simulink model "PTC_MBDS_TurnOnDelaySample_Sample"  (R2013a)
settings: Solver=FixedStepDiscrete  StartTime=0.0  StopTime=100  FixedStep=Auto  RelTol=1e-3
undefined symbols (not defined in the file): sigbuilder_block
libraries: simulink_extras x1, PTC_MBDS_LIB x1
settings Model: Creator=uidl7367  LastModifiedBy=sundeep.tuteja
settings DataIOCC: SignalLoggingSaveFormat=ModelDataLogs
settings OptimizationCC: ExpressionDepthLimit=2147483647  InitFltsAndDblsToZero=on
settings DebuggingCC: SaveWithParameterizedLinksMsg=none  SignalResolutionControl=TryResolveAllWithWarning  SolverPrmCheckMsg=none  InheritedTsInSrcMsg=none  MultiTaskDSMMsg=warning  MultiTaskCondExecSysMsg=none  FcnCallInpInsideContextMsg=UseLocalSettings  StrictBusMsg=Warning
settings RTWCC: IncludeERTFirstTime=on
settings GRTTargetCC: TargetFcnLib=ansi_tfl_tmw.mat  CombineOutputUpdateFcns=off  GRTInterface=on

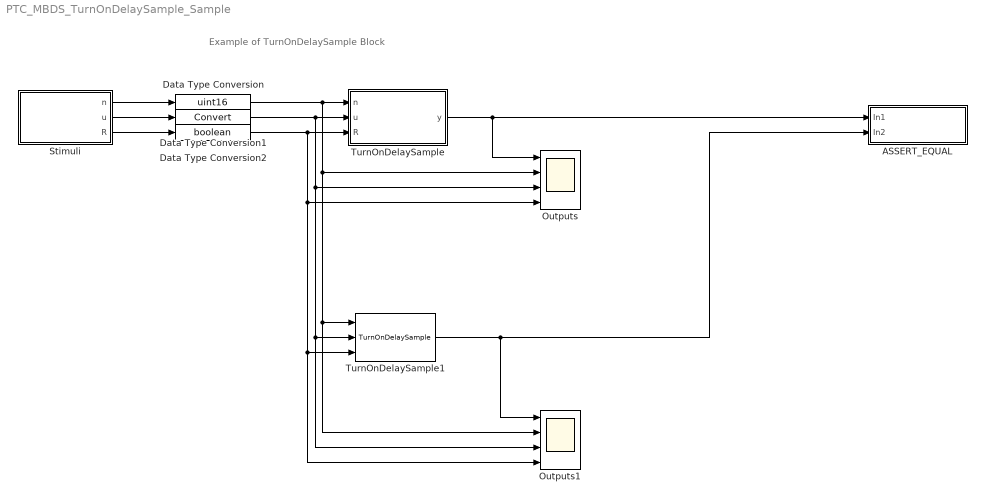
== system PTC_MBDS_TurnOnDelaySample_Sample ==
  note: Example of TurnOnDelaySample Block
  ASSERT_EQUAL : Subsystem
  Data Type Conversion : DataTypeConversion  InitFcn=|  OutDataTypeStr=uint16  SaturateOnIntegerOverflow=on
      | try
      |    MBDS_BlockCallback('Update', gcb);
      | end
  Data Type Conversion1 : DataTypeConversion  InitFcn=|  SaturateOnIntegerOverflow=on
      | try
      |    MBDS_BlockCallback('Update', gcb);
      | end
  Data Type Conversion2 : DataTypeConversion  InitFcn=|  OutDataTypeStr=boolean  SaturateOnIntegerOverflow=on
      | try
      |    MBDS_BlockCallback('Update', gcb);
      | end
  Outputs : Scope  NumInputPorts=4
      settings: TimeRange=100  YMin=0~1~0~0  YMax=1~3~1~1  SampleInput=on  SampleTime=1
  Outputs1 : Scope  NumInputPorts=4
      settings: TimeRange=100  YMin=0~1~0~0  YMax=1~3~1~1  SampleInput=on  SampleTime=1
  Stimuli : Subsystem  Tag=STV Subsys  LoadFcn=sigbuilder_block('load');  StartFcn=sigbuilder_block('start');  StopFcn=sigbuilder_block('stop');  ClipboardFcn=sigbuilder_block('clipboard');  mask(Sigbuilder block){}
      mask help: Sigbuilder GUI
      mask init:
      | if ~strcmp(get_param(bdroot(gcb),'SimulationStatus'),'stopped') tuvar = sigbuilder_block('maskInit'); end
      settings: CopyFcn=sigbuilder_block('copy');  DeleteFcn=sigbuilder_block('delete');  ModelCloseFcn=sigbuilder_block('modelClose');  PreSaveFcn=sigbuilder_block('preSave');  PauseFcn=sigbuilder_block('pause')  ContinueFcn=sigbuilder_block('continue')  NameChangeFcn=sigbuilder_block('namechange');  OpenFcn=sigbuilder_block('open',[0.75 280.5 730.5 239.25 ]);  CloseFcn=sigbuilder_block('close');
      mask Display: plot(0,0,100,100,[10,10,40,40,10],[80,20,20,80,80],[40,10],[50,50], [40,27,10],[65,72,56],[40,25,25,10],[28,28,43,43]);
  TurnOnDelaySample : Subsystem  InitFcn=|  mask(TurnOnDelaySample){MBDS_LibraryBlock=on, R_Enabled=on, IV_Enabled=on, IV=0, MBDS_BlockVersion=05.40}
      | if(exist('MBDS_BlockCallback', 'file'))
      |    MBDS_BlockCallback('Update', gcb);
      | end
      mask prompts: MBDS_LibraryBlock "MBDS library block"; R_Enabled "Show R port"; IV_Enabled "Show IV port"; IV "Init value (IV):"; MBDS_BlockVersion "Block version:"
      mask help: A rising edge of the input signal u is delayed by n block evaluations.
      mask init:
      | if(exist('MBDS_BlockCallback', 'file'))
      |    MBDS_BlockCallback('Init', gcb);
      | else
      |    % Disable all mask parameters
      |    MaskEnables = get_param(gcb, 'MaskEnables');
      |    for k = [1:length(MaskEnables)]
      |       MaskEnables{k} = 'off';
      |    end
      |    if(~isequal(MaskEnables, get_param(gcb, 'MaskEnables')))
      |       set_param(gcb, 'MaskEnables', MaskEnables);
      |    end
      | end
      mask Help: eval(['open([workdir(''library_dir:''),''\Blockset\help\'',get_param(gcb,''MaskType''),''.html''])'])
      mask Callback R_Enabled:
      | % Update mask parameter dialog
      | if(exist('MBDS_BlockCallback', 'file'))
      |    MBDS_BlockCallback('R_Enabled', gcb);
      | end
      mask Display:
      | % Show icon or block text
      | if(exist('TurnOnDelaySample.tif', 'file'))
      |    image(imread('TurnOnDelaySample.tif','tif'), [0.295739348370927 0.17 0.378947368421053 0.66]);
      |    disp('')
      | else
      |    disp(sprintf('Turn-On\nDelay\nSample'));
      | end
      | 
      | % Display port labels
      | port_label('input', 1, 'n');
      | port_label('input', 2, 'u');
      | port_label('input', 3, 'R');
      | port_label('output', 1, 'y');
  TurnOnDelaySample1 : PTC_MBDS_LIB/MBDS Standard Library/Extended Operations/Delay Blocks/TurnOnDelaySample  R_Enabled=on  PTC_MBDS_BlockVersion=5.32  PTC_BlockType=PTC_MBDS_TurnOnDelaySample
  wires:
  Data Type Conversion/1 -> TurnOnDelaySample/1(n), TurnOnDelaySample1/1, Outputs1/2, Outputs/2
  Data Type Conversion1/1 -> TurnOnDelaySample/2(u), TurnOnDelaySample1/2, Outputs1/3, Outputs/3
  Data Type Conversion2/1 -> TurnOnDelaySample/3(R), TurnOnDelaySample1/3, Outputs1/4, Outputs/4
  TurnOnDelaySample/1(y) -> ASSERT_EQUAL/1(In1), Outputs/1
  Stimuli/3(R) -> Data Type Conversion2/1
  Stimuli/2(u) -> Data Type Conversion1/1
  Stimuli/1(n) -> Data Type Conversion/1
  TurnOnDelaySample1/1 -> ASSERT_EQUAL/2(In2), Outputs1/1

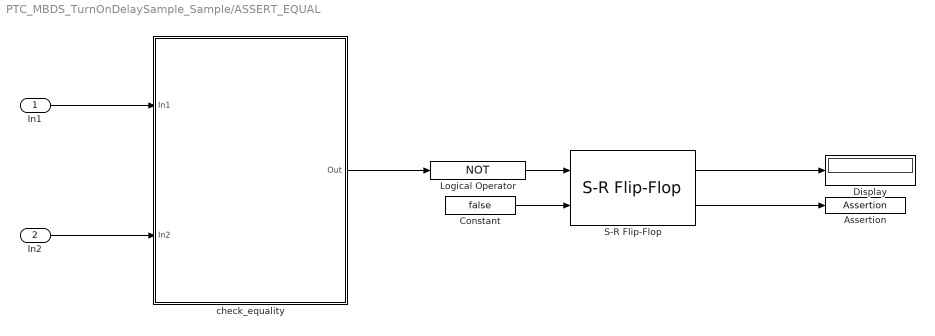
== system PTC_MBDS_TurnOnDelaySample_Sample/ASSERT_EQUAL ==
  In1 : Inport
  In2 : Inport  Port=2
  Assertion : Assertion
  Constant : Constant  Value=false
  Display : Display
  Logical Operator : Logic  Operator=NOT  AllPortsSameDT=off  OutDataTypeStr=boolean
  S-R Flip-Flop : simulink_extras/Flip Flops/S-R Flip-Flop  initial_condition=0
  check_equality : MATLAB Function  TreatAsAtomicUnit=on
  wires:
  S-R Flip-Flop/1 -> Display/1
  check_equality/1(Out) -> Logical Operator/1
  Constant/1 -> S-R Flip-Flop/2
  S-R Flip-Flop/2 -> Assertion/1
  In2/1 -> check_equality/2(In2)
  In1/1 -> check_equality/1(In1)
  Logical Operator/1 -> S-R Flip-Flop/1

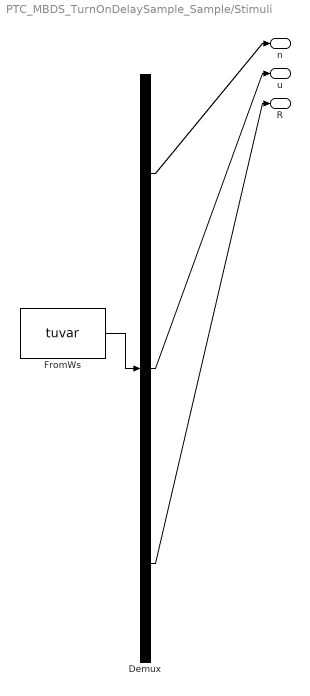
== system PTC_MBDS_TurnOnDelaySample_Sample/Stimuli ==
  Demux : Demux  Tag=STV Demux  Outputs=3
  FromWs : FromWorkspace  Tag=STV FromWs  VariableName=tuvar  SampleTime=0  OutputAfterFinalValue=Holding final value
      SigBuilderData=|
      | common.afterFinalStr = 'Hold final value'
      | common.sampleTime = 0
      | dataSet.timeRange = [0 100]
      | dataSet.name = 'test data'
      | sbobj.Groups.Name = 'test data'
      | sbobj.Groups.Signals(1).Name = 'n'
      | sbobj.Groups.Signals(1).XData = [0 20 20 30 30 100]
      | sbobj.Groups.Signals(1).YData = [1 1 2 2 3 3]
      | sbobj.Groups.Signals(2).Name = 'u'
      | sbobj.Groups.Signals(2).XData = [0 60 60 70 70 100]
      | sbobj.Groups.Signals(2).YData = [0 0 1 1 0 0]
      | sbobj.Groups.Signals(3).Name = 'R'
      | sbobj.Groups.Signals(3).XData = [0 9.5 9.5 10.5 10.5 19.5 19.5 20.5 20.5 29.5 29.5 30.5 30.5 39.5 39.5 40.5 40.5 49.5 49.5 50.5 50.5 80 80 90 90 100]
      | sbobj.Groups.Signals(3).YData = [0 0 1 1 0 0 1 1 0 0 1 1 0 0 1 1 0 0 1 1 0 0 1 1 0 0]
      | sbobj.Groups.TimeRange = [0 100]
  n : Outport  Tag=STV Outport
  u : Outport  Tag=STV Outport  Port=2
  R : Outport  Tag=STV Outport  Port=3
  wires:
  Demux/3 -> R/1
  Demux/2 -> u/1
  Demux/1 -> n/1
  FromWs/1 -> Demux/1

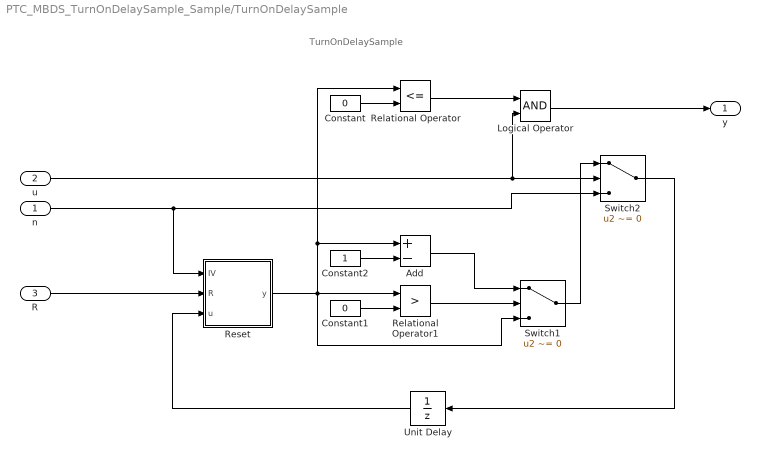
== system PTC_MBDS_TurnOnDelaySample_Sample/TurnOnDelaySample ==
  note: TurnOnDelaySample
  n : Inport
  u : Inport  Port=2
  R : Inport  Port=3  OutDataTypeStr=boolean
  Add : Sum  Inputs=+-  OutDataTypeStr=Inherit: Inherit via back propagation  SaturateOnIntegerOverflow=on
  Constant : Constant  Value=0  OutDataTypeStr=Inherit: Inherit via back propagation
  Constant1 : Constant  Value=0  OutDataTypeStr=Inherit: Inherit via back propagation
  Constant2 : Constant  OutDataTypeStr=Inherit: Inherit via back propagation
  Logical Operator : Logic  OutDataTypeStr=boolean
  Relational Operator : RelationalOperator  Operator=<=  OutDataTypeStr=boolean  InputSameDT=on
  Relational Operator1 : RelationalOperator  Operator=>  OutDataTypeStr=boolean  InputSameDT=on
  Reset : Subsystem
  Switch1 : Switch  Criteria=u2 ~= 0  OutDataTypeStr=Inherit: Inherit via back propagation
  Switch2 : Switch  Criteria=u2 ~= 0  OutDataTypeStr=Inherit: Inherit via back propagation
  Unit Delay : UnitDelay  SampleTime=-1
  y : Outport
  wires:
  Add/1 -> Switch1/1
  Unit Delay/1 -> Reset/3(u)
  Logical Operator/1 -> y/1
  n/1 -> Switch2/3, Reset/1(IV)
  Constant/1 -> Relational Operator/2
  Constant1/1 -> Relational Operator1/2
  Reset/1(y) -> Switch1/3, Relational Operator/1, Add/1, Relational Operator1/1
  Relational Operator1/1 -> Switch1/2
  Relational Operator/1 -> Logical Operator/1
  Switch2/1 -> Unit Delay/1
  Constant2/1 -> Add/2
  u/1 -> Logical Operator/2, Switch2/2
  Switch1/1 -> Switch2/1
  R/1 -> Reset/2(R)

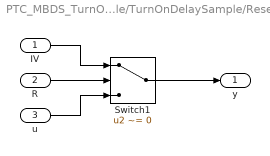
== system PTC_MBDS_TurnOnDelaySample_Sample/TurnOnDelaySample/Reset ==
  IV : Inport
  R : Inport  Port=2
  u : Inport  Port=3
  Switch1 : Switch  Criteria=u2 ~= 0  OutDataTypeStr=Inherit: Inherit via back propagation  InputSameDT=on
  y : Outport
  wires:
  u/1 -> Switch1/3
  Switch1/1 -> y/1
  IV/1 -> Switch1/1
  R/1 -> Switch1/2

== matlab function PTC_MBDS_TurnOnDelaySample_Sample/ASSERT_EQUAL/check_equality ==
  data: In1 input; Out output; In2 input
function Out = check_equality(In1, In2)
%#codegen

Out = isequaln(In1, In2);

end
